simulink model "bicycle_model"  (R2023b)
settings: Solver=ode4  StartTime=0.0  StopTime=3  FixedStep=0.01  MaxStep=0.2  RelTol=1e-3
undefined symbols (not defined in the file): A, B, C, D, K
settings Model: Creator=11935  LastModifiedBy=11935

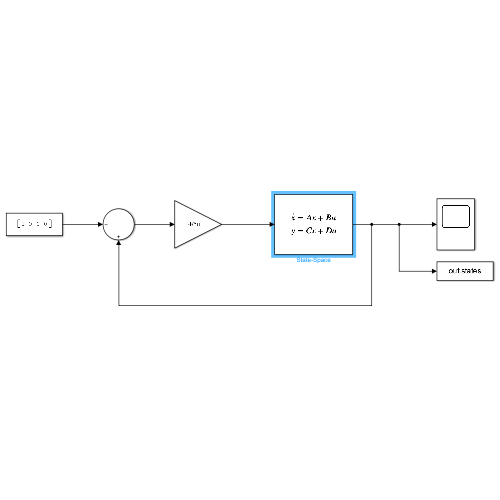
[thumbnail: Simulink's stored preview of the top-level diagram]
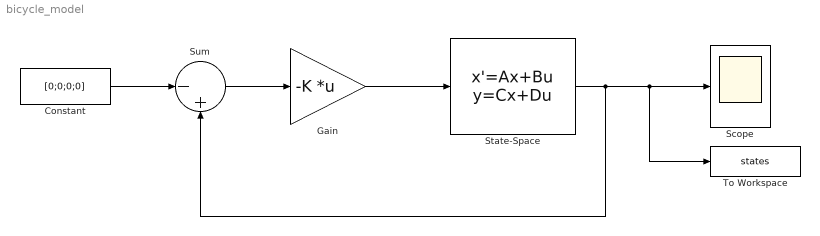
== system bicycle_model ==
  Constant : Constant  Value=[0;0;0;0]
  Gain : Gain  Gain=-K  Multiplication=Matrix(K*u)
  Scope : Scope
  State-Space : StateSpace  A=A  B=B  C=C  D=D  InitialCondition=[0.5;0;0.1;0]
  Sum : Sum  Inputs=|-+
  To Workspace : ToWorkspace  VariableName=states  SaveFormat=Structure With Time  SampleTime=-1
  wires:
  Constant/1 -> Sum/1
  Sum/1 -> Gain/1
  Gain/1 -> State-Space/1
  State-Space/1 -> Scope/1, To Workspace/1, Sum/2
